simulink model "TF_SingleDof_2018a"  (R2018a)
settings: Solver=FixedStepAuto  StartTime=0.0  StopTime=60  FixedStep=0.001  RelTol=1e-3
values from neighbouring files (symbols this model uses):
  c = 4    [MakeSomeNoise.m]
  k = 10    [MakeSomeNoise.m]
  m = 3    [MakeSomeNoise.m]
settings Model: Creator=dongxh  LastModifiedBy=dongxh
settings DataIOCC: ReturnWorkspaceOutputs=on
settings DebuggingCC: UnconnectedInputMsg=none  UnconnectedOutputMsg=none  UnconnectedLineMsg=none  SFMachineParentedDataDiag=error
settings ModelReferenceCC: EnableRefExpFcnMdlSchedulingChecks=off
settings SFSimCC: SimUseLocalCustomCode=on
settings RTWCC: Description=Generic Real-Time Target  RTWUseLocalCustomCode=on

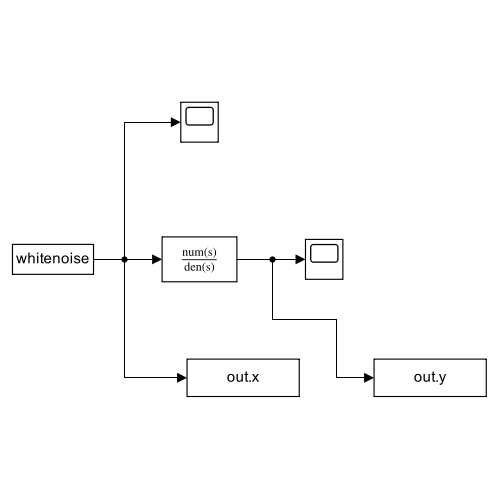
[thumbnail: Simulink's stored preview of the top-level diagram]
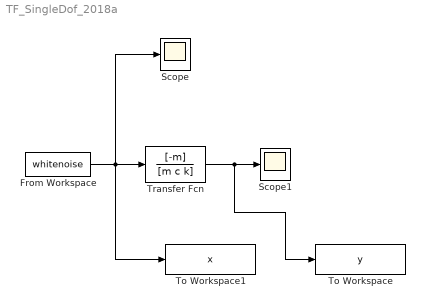
== system TF_SingleDof_2018a ==
  From Workspace : FromWorkspace  VariableName=whitenoise  SampleTime=-1
  Scope : Scope
  Scope1 : Scope
  To Workspace : ToWorkspace  VariableName=y  SampleTime=-1
      settings: Save2DSignal=2-D array (concatenate along first dimension)
  To Workspace1 : ToWorkspace  VariableName=x  SampleTime=-1
      settings: Save2DSignal=2-D array (concatenate along first dimension)
  Transfer Fcn : TransferFcn  Numerator=[-m]  Denominator=[m c k]
  wires:
  From Workspace/1 -> Scope/1, To Workspace1/1, Transfer Fcn/1
  Transfer Fcn/1 -> To Workspace/1, Scope1/1
